simulink model "Static_Deflection_State_Space"  (R2014a)
settings: Solver=ode23t  StartTime=0.0  StopTime=100  RelTol=1e-3
InitFcn:
  | %if ~exist('linsys_beam_fixfree','var') ||~exist('linsys_beam_rotfree','var')
  |    load SS_Damping_1e7.mat
  |    disp('State Space Models does not exist in workspace, loading presaved SS models')
  | %end
StopFcn:
  | disp(['Static Deflection is ' num2str(SS_Def.signals.values(end)) ' m'])
undefined symbols (not defined in the file): beam_wall, beam_width, density, element_length, gravity, num_elem
libraries: cstblocks x1
Description:
  | Copyright 2014 The MathWorks, Inc.
settings Model: Creator=psanghvi  LastModifiedBy=smiller
settings DebuggingCC: UnderspecifiedInitializationDetection=Classic

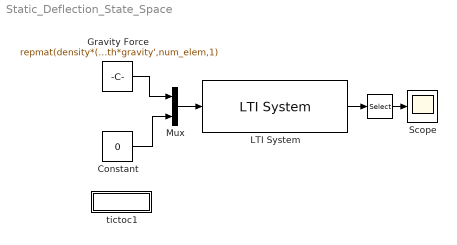
== system Static_Deflection_State_Space ==
  "  " : Selector  InputPortWidth=num_elem+1  Indices=num_elem+1
  Constant : Constant  Value=0
  Gravity Force : Constant  Value=repmat(density*(beam_width^2- (beam_width-beam_wall*2)^2)*element_length*gravity',num_elem,1)
  LTI System : cstblocks/LTI System  sys=linsys_beam_fixfree  IC=[]
  Mux : Mux  Inputs=2
  Scope : Scope
      settings: YMin=-2  YMax=0  SaveName=SS_Def
  tictoc1 : Subsystem
      settings: OpenFcn=open('Flexible_Beam_Demo_Script.html')
      mask Display: disp('Script')
  wires:
  Constant/1 -> Mux/2
  Gravity Force/1 -> Mux/1
  Mux/1 -> LTI System/1
  LTI System/1 -> "  "/1
  "  "/1 -> Scope/1

== system Static_Deflection_State_Space/tictoc1 ==
